simulink model "tutorial1"  (R2023b)
settings: Solver=ode45  StartTime=0.0  StopTime=20  MaxStep=1e-3  RelTol=1e-3
settings Model: Creator=izabe  LastModifiedBy=izabe

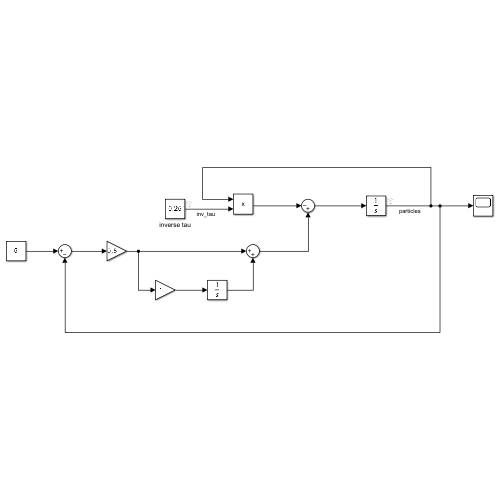
[thumbnail: Simulink's stored preview of the top-level diagram]
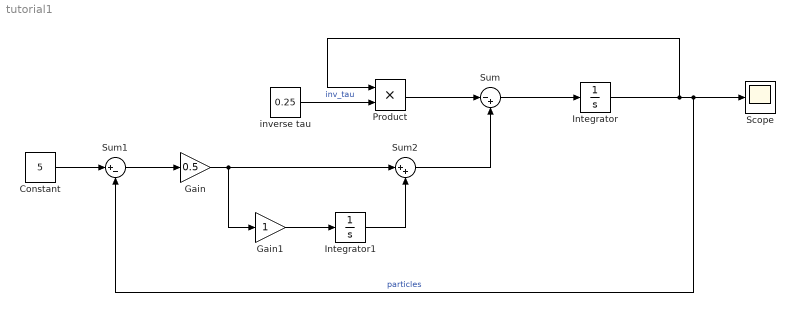
== system tutorial1 ==
  Constant : Constant  Value=5
  Gain : Gain  Gain=0.5
  Gain1 : Gain
  Integrator : Integrator
  Integrator1 : Integrator
  Product : Product
  Scope : Scope
  Sum : Sum  Inputs=|-+
  Sum1 : Sum  Inputs=|+-
  Sum2 : Sum  Inputs=|++
  inverse tau : Constant  Value=0.25
  wires:
  inverse tau/1 -> Product/2  "inv_tau"
  Product/1 -> Sum/1
  Sum/1 -> Integrator/1
  Integrator/1 -> Product/1, Sum1/2, Scope/1  "particles"
  Constant/1 -> Sum1/1
  Sum1/1 -> Gain/1
  Gain/1 -> Gain1/1, Sum2/1
  Integrator1/1 -> Sum2/2
  Sum2/1 -> Sum/2
  Gain1/1 -> Integrator1/1
